simulink model "Demo1_model"  (R2024a)
settings: Solver=VariableStepAuto  StartTime=0.0  StopTime=1  RelTol=1e-3
libraries: commchan3 x2, simulink x2, commcnvcod2 x2, dspvision x2, commdigbbndpm3 x2, commfilt2 x2, commsink2 x1, commutil2 x1, dspindex x1
settings Model: Creator=joeji  LastModifiedBy=Q
settings OptimizationCC: BlockReduction=off  ConditionallyExecuteInputs=off

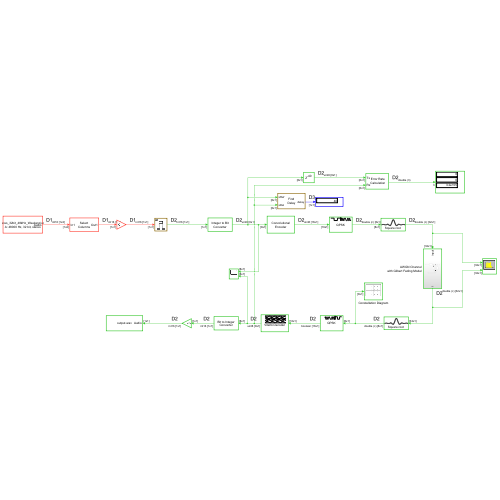
[thumbnail: Simulink's stored preview of the top-level diagram]
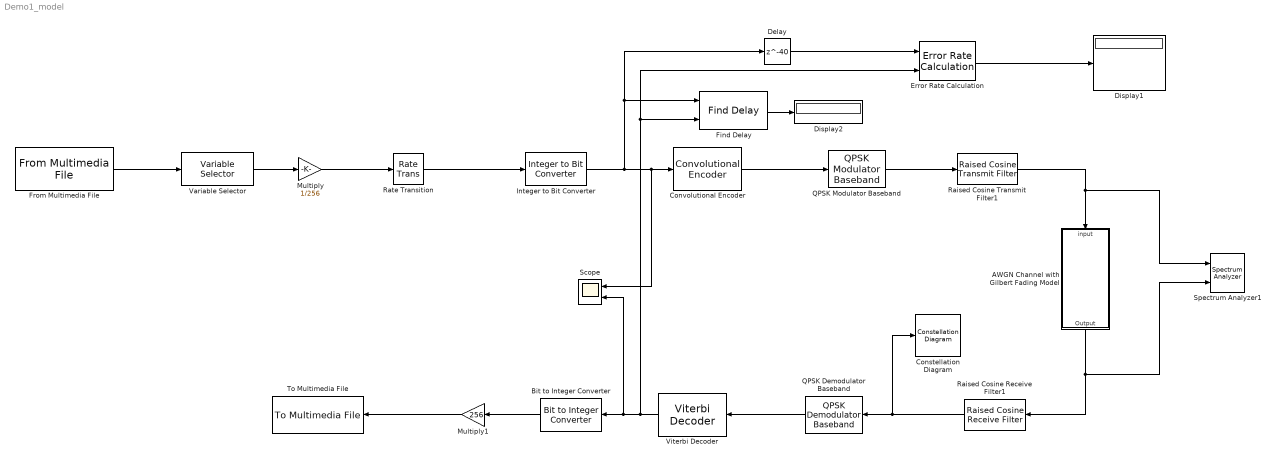
== system Demo1_model ==
  AWGN Channel with Gilbert Fading Model : Subsystem
  Bit to Integer Converter : simulink/Logic and Bit Operations/Bit to Integer Converter  nbits=8  bitOrder=MSB first  signedOutputValues=Signed  outDtype=Inherit via internal rule  outDtypeSigned=int16
      settings: LibrarySourceBlock=|
      | commutil2/Bit to Integer
      | Converter
  Constellation Diagram : ConstellationDiagram  WindowPosition=[193.000000,61.000000,600.000000,600.000000,]  Visible=on  ScopeFrameLocation=window
  Convolutional Encoder : commcnvcod2/Convolutional Encoder  trellis=poly2trellis(7, [171 133])  opMode=Continuous  DelayedResetAction=on  hasIniStPort=off  hasFinStPort=off  usePuncVector=off  punctureVector=[1; 1; 0; 1; 0; 1]  reset=Unused parameter value
      settings: LibrarySourceBlock=|
      | commhdlcnvcod/Convolutional
      | Encoder
  Delay : Delay  DelayLength=40  InputProcessing=Columns as channels (frame based)
  Display1 : Display
  Display2 : Display
  Error Rate Calculation : commsink2/Error Rate Calculation  N=0  st_delay=2  cp_mode=Entire frame  subframe=[]  PMode=Port  WsName=ErrorVec  RsMode2=off  stop=off  numErr=100  maxBits=1e6
      settings: LibrarySourceBlock=|
      | commhdlsink/Error Rate
      | Calculation
  Find Delay : commutil2/Find Delay  corrLength=200  chgSigOP=off  stopUpdate=on  numConstDelay=3
  From Multimedia File : dspvision/From Multimedia File  inputFilename=D:\ubc\UBC_4th\ELEC 391\Sound_file\Stereo_32bit_48kHz_Weekend.wav  readRange=[1 Inf]  loop=on  numPlays=inf  outputStreams=Audio only  videoDataType=single  audioDataType=int16  inheritSampleTime=on  userDefinedSampleTime=1/30  noAudioOutput=off  isIntensityVideo=off  fourcc=RGB  colorVideoFormat=Separate color signals  outputEOF=off  dataOrg=Column-major  audioFrameSize=1  computeAudioFrameSize=off  outSamplingMode=Sample based
      settings: LibrarySourceBlock=audiosources/From Multimedia File
  Integer to Bit Converter : simulink/Logic and Bit Operations/Integer to Bit Converter  nbits=8  signedInputValues=Signed  bitOrder=MSB first  outDtype=uint8
  Multiply : Gain  Gain=1/256  OutDataTypeStr=int16
  Multiply1 : Gain  Gain=256  OutDataTypeStr=int16
  QPSK Demodulator Baseband : commdigbbndpm3/QPSK Demodulator Baseband  OutType=Bit  DecType=Hard decision  VarSource=Dialog  Variance=1  Dec=Gray  Ph=pi/4  outDtype1=boolean  outDtype2=Inherit via internal rule  derotateFactorWordLen=16  derotateFactorDataTypeStr=Inherit: Same word length as input  derotateFactorLastDataTypeStr=Inherit: Same word length as input
  QPSK Modulator Baseband : commdigbbndpm3/QPSK Modulator Baseband  InType=Bit  Enc=Gray  Ph=pi/4  outDtype=double  outWordLen=16  outUDDataType=sfix(16)  outFracLenMode=Best precision  outFracLen=15  outDataTypeStr=double  outLastDataTypeStr=double
  Raised Cosine Receive Filter1 : commfilt2/Raised Cosine Receive Filter  filtType=Square root  R=0.5  filtSpan=8  N=4  downFactor=4  downOffset=0  filterGain=1  InputProcessing=Columns as channels (frame based)  RateOptions=Enforce single-rate processing  framing=Mute  checkCoeff=off  variableName=rcRxFilt1  currentFiltSpan=10  D=5  inputOffset=0  sampMode=Mute  saveAsFlag=0  rateMode=Downsampling  checkGain=Normalized  launchFVT=on  roundingMode=Floor  overflowMode=off  coeffDataTypeStr=Inherit: Same word length as input  coeffMin=[]  coeffMax=[]  coeffLastDataTypeStr=Inherit: Same word length as input  accumDataTypeStr=Inherit: Same as product output  accumLastDataTypeStr=Inherit: Same as product output  outputDataTypeStr=Inherit: Same as accumulator  outputMin=[]  outputMax=[]  outputLastDataTypeStr=Inherit: Same as accumulator
  Raised Cosine Transmit Filter1 : commfilt2/Raised Cosine Transmit Filter  filtType=Square root  R=0.5  filtSpan=8  N=4  filterGain=1  InputProcessing=Columns as channels (frame based)  RateOptions=Enforce single-rate processing  framing=Mute  checkCoeff=off  variableName=rcTxFilt1  checkGain=Normalized  sampMode=Mute  saveAsFlag=0  currentFiltSpan=10  D=(10)/2  launchFVT=on  roundingMode=Floor  overflowMode=off  coeffDataTypeStr=Inherit: Same word length as input  coeffMin=[]  coeffMax=[]  coeffLastDataTypeStr=Inherit: Same word length as input  outputDataTypeStr=Inherit: Same as accumulator  outputMin=[]  outputMax=[]  outputLastDataTypeStr=Inherit: Same as accumulator
  Rate Transition : RateTransition  Integrity=off  OutPortSampleTime=1/40000
  Scope : Scope  NumInputPorts=2
  Spectrum Analyzer1 : SpectrumAnalyzer  NumInputPorts=2  WindowPosition=[0.000000,32.000000,1536.000000,800.000000,]  Visible=on  ScopeFrameLocation=window  PlotAsTwoSidedSpectrum=off  FrequencySpan=Start and stop frequencies  Span=2520000  CenterFrequency=1260000  StartFrequency=0  StopFrequency=500000  YLimits=[-108.30431803,21.18944778]  ShowLegend=on
  To Multimedia File : dspvision/To Multimedia File  outputFilename=D:\ubc\UBC_4th\ELEC 391\Demo1\output.wav  streamSelection=Audio only  videoCompressor=None (uncompressed)  audioCompressor=None (uncompressed)  imagePorts=One multidimensional signal  fileType=WAV  audioDatatype=16-bit integer  fourcc=RGB  audioBitRate=128  audioQuality=75  videoQuality=75  mj2000CompFactor=10
      settings: LibrarySourceBlock=dspsnks4/To Multimedia File
  Variable Selector : dspindex/Variable Selector  NumInputs=1  rowsOrCols=Columns  IdxMode=Fixed  Elements=[1]  ZerOneIdxMode=One-based  errmode=Clip Index  FillMode=on  FillValues=0
  Viterbi Decoder : commcnvcod2/Viterbi Decoder  trellis=poly2trellis(7, [171 133])  isPunctured=off  punctureVector=[1; 1; 0; 1; 0; 1]  erasures=off  dectype=Hard decision  nsdecb=4  runSigValErrCheck=off  tbdepth=32  opmode=Continuous  reset=off  delayedResetAction=on  smWordLength=16  outDataType=Smallest unsigned integer
      settings: LibrarySourceBlock=commhdlcnvcod/Viterbi Decoder
  wires:
  QPSK Modulator Baseband/1 -> Raised Cosine Transmit Filter1/1
  Integer to Bit Converter/1 -> Delay/1, Find Delay/1, Convolutional Encoder/1, Scope/1
  Error Rate Calculation/1 -> Display1/1
  Delay/1 -> Error Rate Calculation/1
  Variable Selector/1 -> Multiply/1
  From Multimedia File/1 -> Variable Selector/1
  Raised Cosine Transmit Filter1/1 -> AWGN Channel with Gilbert Fading Model/1(input), Spectrum Analyzer1/1
  Raised Cosine Receive Filter1/1 -> QPSK Demodulator Baseband/1, Constellation Diagram/1
  Viterbi Decoder/1 -> Find Delay/2, Error Rate Calculation/2, Scope/2, Bit to Integer Converter/1
  Rate Transition/1 -> Integer to Bit Converter/1
  Bit to Integer Converter/1 -> Multiply1/1
  Multiply1/1 -> To Multimedia File/1
  Multiply/1 -> Rate Transition/1
  Find Delay/1 -> Display2/1
  QPSK Demodulator Baseband/1 -> Viterbi Decoder/1
  AWGN Channel with Gilbert Fading Model/1(Output) -> Spectrum Analyzer1/2, Raised Cosine Receive Filter1/1
  Convolutional Encoder/1 -> QPSK Modulator Baseband/1

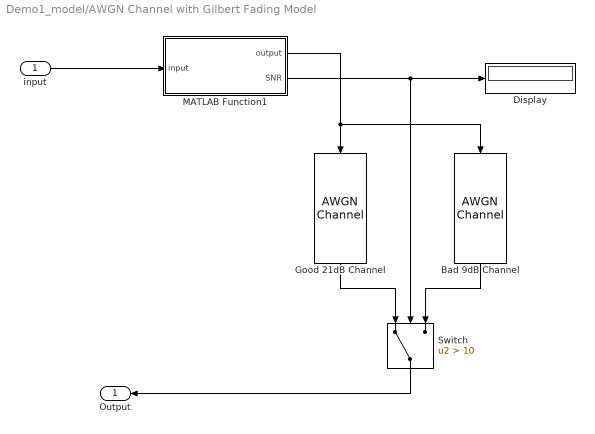
== system Demo1_model/AWGN Channel with Gilbert Fading Model ==
  input : Inport
  Bad 9dB Channel : commchan3/AWGN Channel  LegacyMode=off  NoiseMethod="Signal to noise ratio  (SNR)"  noiseMode="Signal to noise ratio  (SNR)"  EbNo=10  EsNo=10  SNR=9  BitsPerSymbol=1  SignalPower=1  SamplesPerSymbol=1  SymbolPeriod=1  VarianceSource=Parameter  Variance=1  RandomStream=Global stream  Seed=67  SimulateUsing=Code generation
  Display : Display
  Good 21dB Channel : commchan3/AWGN Channel  LegacyMode=off  NoiseMethod="Signal to noise ratio  (SNR)"  noiseMode="Signal to noise ratio  (SNR)"  EbNo=10  EsNo=10  SNR=21  BitsPerSymbol=1  SignalPower=1  SamplesPerSymbol=1  SymbolPeriod=1  VarianceSource=Parameter  Variance=1  RandomStream=Global stream  Seed=67  SimulateUsing=Code generation
  MATLAB Function1 : MATLAB Function  TreatAsAtomicUnit=on
  Switch : Switch  Criteria=u2 > Threshold  Threshold=10  SaturateOnIntegerOverflow=off  InputSameDT=off
  Output : Outport
  wires:
  MATLAB Function1/1(output) -> Good 21dB Channel/1, Bad 9dB Channel/1
  MATLAB Function1/2(SNR) -> Switch/2, Display/1
  Good 21dB Channel/1 -> Switch/1
  Switch/1 -> Output/1
  Bad 9dB Channel/1 -> Switch/3
  input/1 -> MATLAB Function1/1(input)

== matlab function Demo1_model/AWGN Channel with Gilbert Fading Model/MATLAB Function1 ==
  data: output output; input input; SNR output
function [output, SNR] = Gilbert(input)
% Scenario F Gilbert Model Parameters
P_GB = 0.03; % Increased transition probability from Good to Bad
P_BG = 0.25; % Decreased transition probability from Bad to Good
f_tr = 10e3; % State transition frequency in Hz
Ts = 1 / f_tr; % Sampling time

persistent state count;
if isempty(state)
    state = 'G'; % Initial state is Good
    count = 0;
end

% Update count
count = count + 1;

% Gilbert model logic with state transition frequency
if count >= Ts
    count = 0; % Reset count after each time step
    if strcmp(state, 'G')
        if rand < P_GB
            state = 'B';
        end
    else
        if rand < P_BG
            state = 'G';
        end
    end
end

% Determine current state
if strcmp(state, 'G')
    SNR = 21;
else
    SNR = 9;
end

% Output the unchanged input signal
output = input;
